simulink model "BBB_Gyro_Test_LibraryBlock"  (R2013a)
settings: Solver=FixedStepDiscrete  StartTime=0.0  StopTime=inf  FixedStep=0.01  RelTol=1e-3
libraries: BLACKlink x1
settings Model: SimulationMode=external  ExtModeTrigDuration=100  Creator=rdustinkahawita  LastModifiedBy=rdustinkahawita
settings OptimizationCC: OptimizeModelRefInitCode=on  LifeSpan=1
settings DebuggingCC: SolverPrmCheckMsg=none  StrictBusMsg=Warning
settings HardwareCC: ProdLargestAtomicInteger=Long  ProdLargestAtomicFloat=Double  ProdEndianess=LittleEndian  ProdHWDeviceType=ARM Compatible->ARM Cortex
settings RTWCC: SystemTargetFile=realtime.tlc  GenerateMakefile=off  TemplateMakefile=realtime.tmf  Description=Run on Target Hardware  RTWVerbose=off  ProcessScript=realtime_make_rtw_hook
settings STFCustomTargetCC: TargetLibSuffix=.a  GenerateSampleERTMain=on  ERTCustomFileBanners=on  SupportNonInlinedSFcns=off  SupportVariableSizeSignals=on  MATLABClassNameForMDSCustomization=Simulink.SoftwareTarget.ERTCustomization  SystemTargetFile=realtime.tlc
settings ERTTargetCC: ParMdlRefBuildCompliant=off  CompOptLevelCompliant=off  ConcurrentExecutionCompliant=off  CombineOutputUpdateFcns=off  ERTFirstTimeCompliant=off  SupportContinuousTime=on  SupportVariableSizeSignals=on  ModelStepFunctionPrototypeControlCompliant=off  CPPClassGenCompliant=off  ExtMode=on  ExtModeMexArgs='192.168.7.2' 0 17725  ERTSrcFileBannerTemplate=realtime_code_template.cgt  ERTHdrFileBannerTemplate=realtime_code_template.cgt  ERTDataSrcFileTemplate=realtime_code_template.cgt  ERTDataHdrFileTemplate=realtime_code_template.cgt  ERTCustomFileTemplate=realtime_file_process.tlc

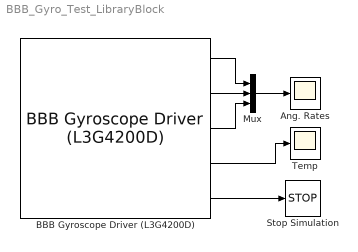
== system BBB_Gyro_Test_LibraryBlock ==
  Ang. Rates : Scope
      settings: TimeRange=30  YMin=-175  YMax=250
  "BBB Gyroscope Driver (L3G4200D) " : BLACKlink/BBB Gyroscope Driver (L3G4200D)   BBB_I2CBus=BeagleBone Black I2C Channel 1  BBB_I2CAddress=Gyro Address: 0x068  BBB_GyroRange=Range: 250 deg/sec  BBB_DebugInfo=Debug Level 0 - Basic Info Only
  Mux : Mux  Inputs=3
  Stop Simulation : Stop
  Temp : Scope
      settings: YMin=16  YMax=16
  wires:
  "BBB Gyroscope Driver (L3G4200D) "/2 -> Mux/2
  "BBB Gyroscope Driver (L3G4200D) "/3 -> Mux/3
  "BBB Gyroscope Driver (L3G4200D) "/4 -> Temp/1
  "BBB Gyroscope Driver (L3G4200D) "/5 -> Stop Simulation/1
  "BBB Gyroscope Driver (L3G4200D) "/1 -> Mux/1
  Mux/1 -> Ang. Rates/1
